simulink model "ControlloRobusto"  (R2021a)
settings: Solver=VariableStepAuto  StartTime=0.0  StopTime=50  RelTol=1e-3
values from neighbouring files (symbols this model uses):
  KD = kdi*eye(4)    [traiettoria.m]
  Kd = 200*diag([1 1 1 1])    [traiettoria.m]
  KP = kpi*eye(4)    [traiettoria.m]
  q0 = scara.ikine(T0, 'mask', [1 1 1 1 0 0])    [pseudo_traiettoria.m]    (also in traiettoria.m)
  Tc = 0.001    [pseudo_traiettoria.m]    (also in traiettoria.m)
undefined symbols (not defined in the file or in its folder): D, DiscIntNeverNeededParam, Kp, Q
settings Model: Creator=Ciro  LastModifiedBy=Ciro

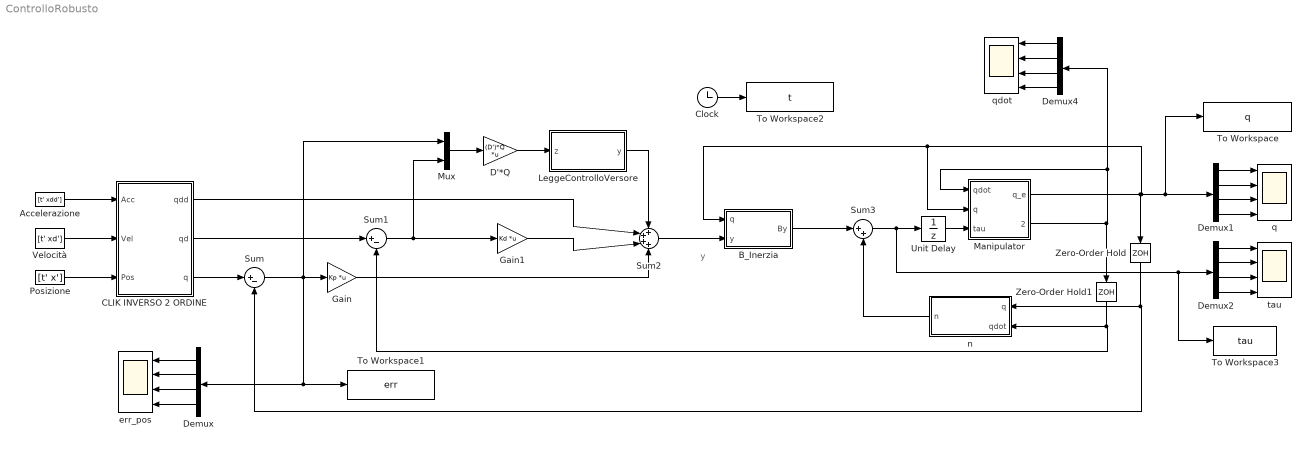
== system ControlloRobusto ==
  note: y
  Accelerazione : FromWorkspace  VariableName=[t' xdd']  SampleTime=Tc  OutputAfterFinalValue=Holding final value
  B_Inerzia : MATLAB Function  TreatAsAtomicUnit=on
  CLIK INVERSO 2 ORDINE : Subsystem
  Clock : Clock
  D'*Q : Gain  Gain=(D')*Q  Multiplication=Matrix(K*u)
  Demux{,1..2,4} (4 alike) : Demux
  Gain : Gain  Gain=Kp  Multiplication=Matrix(K*u)
  Gain1 : Gain  Gain=Kd  Multiplication=Matrix(K*u)
  LeggeControlloVersore : MATLAB Function  TreatAsAtomicUnit=on
  Manipulator : Subsystem
  Mux : Mux  Inputs=2
  Posizione : FromWorkspace  VariableName=[t' x']  SampleTime=Tc  OutputAfterFinalValue=Holding final value
  Sum : Sum  Inputs=|+-
  Sum1 : Sum  Inputs=|+-
  Sum2 : Sum  Inputs=++++
  Sum3 : Sum  Inputs=|++
  To Workspace : ToWorkspace  VariableName=q  SampleTime=-1
      settings: Save2DSignal=2-D array (concatenate along first dimension)
  To Workspace1 : ToWorkspace  VariableName=err  SampleTime=-1
      settings: Save2DSignal=2-D array (concatenate along first dimension)
  To Workspace2 : ToWorkspace  VariableName=t  SampleTime=-1
      settings: Save2DSignal=2-D array (concatenate along first dimension)
  To Workspace3 : ToWorkspace  VariableName=tau  SampleTime=-1
      settings: Save2DSignal=2-D array (concatenate along first dimension)
  Unit Delay : UnitDelay  SampleTime=Tc  HasFrameUpgradeWarning=on
  Velocità : FromWorkspace  VariableName=[t' xd']  SampleTime=Tc  OutputAfterFinalValue=Holding final value
  Zero-Order Hold : ZeroOrderHold  SampleTime=Tc
  Zero-Order Hold1 : ZeroOrderHold  SampleTime=Tc
  err_pos : Scope  NumInputPorts=4
  n : MATLAB Function  TreatAsAtomicUnit=on
  q : Scope  NumInputPorts=4
  qdot : Scope  NumInputPorts=4
  tau : Scope  NumInputPorts=4
  wires:
  Accelerazione/1 -> CLIK INVERSO 2 ORDINE/1(Acc)
  Velocità/1 -> CLIK INVERSO 2 ORDINE/2(Vel)
  Posizione/1 -> CLIK INVERSO 2 ORDINE/3(Pos)
  Sum/1 -> Mux/1, Gain/1, To Workspace1/1, Demux/1
  Sum1/1 -> Mux/2, Gain1/1
  B_Inerzia/1(By) -> Sum3/1
  CLIK INVERSO 2 ORDINE/3(q) -> Sum/1
  CLIK INVERSO 2 ORDINE/2(qd) -> Sum1/1
  n/1(n) -> Sum3/2
  Sum3/1 -> Unit Delay/1, To Workspace3/1, Demux2/1
  Gain1/1 -> Sum2/3
  CLIK INVERSO 2 ORDINE/1(qdd) -> Sum2/2
  Demux/1 -> err_pos/1
  Demux/2 -> err_pos/2
  Demux/3 -> err_pos/3
  Demux/4 -> err_pos/4
  Demux1/1 -> q/1
  Demux1/2 -> q/2
  Demux1/3 -> q/3
  Demux1/4 -> q/4
  Demux2/4 -> tau/4
  Demux2/3 -> tau/3
  Demux2/2 -> tau/2
  Demux2/1 -> tau/1
  LeggeControlloVersore/1(y) -> Sum2/1
  Mux/1 -> D'*Q/1
  D'*Q/1 -> LeggeControlloVersore/1(z)
  Demux4/4 -> qdot/4
  Demux4/3 -> qdot/3
  Demux4/2 -> qdot/2
  Demux4/1 -> qdot/1
  Gain/1 -> Sum2/4
  Manipulator/1(q_e) -> Demux1/1, To Workspace/1, B_Inerzia/1(q), Manipulator/2(q), Zero-Order Hold/1
  Manipulator/2(qdot_e) -> Demux4/1, Manipulator/1(qdot), Zero-Order Hold1/1
  Zero-Order Hold/1 -> Sum/2, n/1(q)
  Zero-Order Hold1/1 -> Sum1/2, n/2(qdot)
  Sum2/1 -> B_Inerzia/2(y)
  Unit Delay/1 -> Manipulator/3(tau)
  Clock/1 -> To Workspace2/1

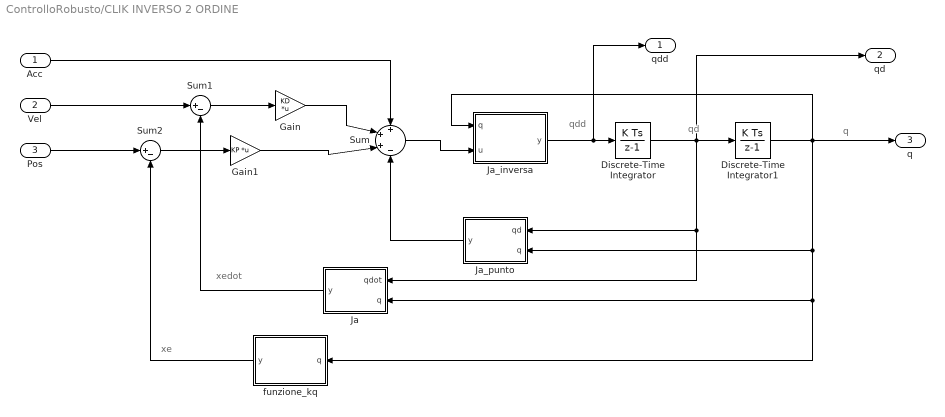
== system ControlloRobusto/CLIK INVERSO 2 ORDINE ==
  note: qdd
  note: xedot
  note: xe
  note: qd
  note: q
  Acc : Inport
  Vel : Inport  Port=2
  Pos : Inport  Port=3
  Discrete-Time Integrator : DiscreteIntegrator  InitialCondition=[0; 0; 0; 0]  SampleTime=Tc  ICPrevOutput=DiscIntNeverNeededParam  ICPrevScaledInput=DiscIntNeverNeededParam
  Discrete-Time Integrator1 : DiscreteIntegrator  InitialCondition=q0  SampleTime=Tc  ICPrevOutput=DiscIntNeverNeededParam  ICPrevScaledInput=DiscIntNeverNeededParam
  Gain : Gain  Gain=KD  Multiplication=Matrix(K*u)
  Gain1 : Gain  Gain=KP  Multiplication=Matrix(K*u)
  Ja : MATLAB Function  TreatAsAtomicUnit=on
  Ja_inversa : MATLAB Function  TreatAsAtomicUnit=on
  Ja_punto : MATLAB Function  TreatAsAtomicUnit=on
  Sum : Sum  Inputs=+++-
  Sum1 : Sum  Inputs=|+-
  Sum2 : Sum  Inputs=|+-
  funzione_kq : MATLAB Function  TreatAsAtomicUnit=on
  qdd : Outport
  qd : Outport  Port=2
  q : Outport  Port=3
  wires:
  Gain1/1 -> Sum/3
  Discrete-Time Integrator1/1 -> q/1, Ja_punto/2(q), Ja/2(q), funzione_kq/1(q), Ja_inversa/1(q)
  Ja_punto/1(y) -> Sum/4
  Pos/1 -> Sum2/1
  Sum/1 -> Ja_inversa/2(u)
  Gain/1 -> Sum/2
  Sum2/1 -> Gain1/1
  funzione_kq/1(y) -> Sum2/2
  Ja/1(y) -> Sum1/2
  Sum1/1 -> Gain/1
  Vel/1 -> Sum1/1
  Acc/1 -> Sum/1
  Discrete-Time Integrator/1 -> qd/1, Ja_punto/1(qd), Ja/1(qdot), Discrete-Time Integrator1/1
  Ja_inversa/1(y) -> qdd/1, Discrete-Time Integrator/1

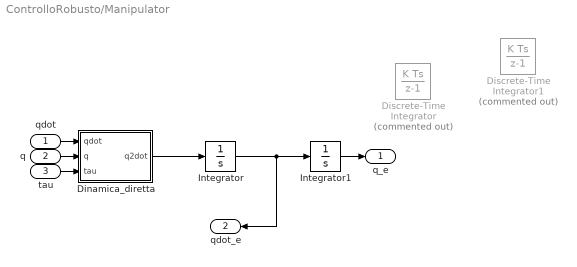
== system ControlloRobusto/Manipulator ==
  qdot : Inport
  q : Inport  Port=2
  tau : Inport  Port=3
  Dinamica_diretta : MATLAB Function  TreatAsAtomicUnit=on
  Discrete-Time Integrator : DiscreteIntegrator  Commented=on  InitialCondition=[0; 0; 0; 0]  SampleTime=Tc  ICPrevOutput=DiscIntNeverNeededParam  ICPrevScaledInput=DiscIntNeverNeededParam
  Discrete-Time Integrator1 : DiscreteIntegrator  Commented=on  InitialCondition=q0  SampleTime=Tc  ICPrevOutput=DiscIntNeverNeededParam  ICPrevScaledInput=DiscIntNeverNeededParam
  Integrator : Integrator  InitialCondition=[0; 0; 0; 0]
  Integrator1 : Integrator  InitialCondition=q0
  q_e : Outport
  qdot_e : Outport  Port=2
  wires:
  tau/1 -> Dinamica_diretta/3(tau)
  qdot/1 -> Dinamica_diretta/1(qdot)
  q/1 -> Dinamica_diretta/2(q)
  Integrator1/1 -> q_e/1
  Integrator/1 -> Integrator1/1, qdot_e/1
  Dinamica_diretta/1(q2dot) -> Integrator/1

== matlab function ControlloRobusto/CLIK INVERSO 2 ORDINE/Ja_inversa ==
  data: q input; u input; y output
function y = fcn(q, u)
J = [ -0.5*(sin(q(1))+sin(q(1)+q(2))) -0.5*sin(q(1)+q(2))  0  0;
       0.5*(cos(q(1))+cos(q(1)+q(2)))  0.5*cos(q(1)+q(2))  0  0;
       0                               0                  -1  0;
       1                               1                   0 -1];
y = inv(J)*u;

== matlab function ControlloRobusto/CLIK INVERSO 2 ORDINE/Ja ==
  data: qdot input; q input; y output
function y = fcn(qdot,q)
J = [ -0.5*(sin(q(1))+sin(q(1)+q(2))) -0.5*sin(q(1)+q(2))  0  0;
       0.5*(cos(q(1))+cos(q(1)+q(2)))  0.5*cos(q(1)+q(2))  0  0;
       0                               0                  -1  0;
       1                               1                   0 -1];
y = J*qdot;

== matlab function ControlloRobusto/CLIK INVERSO 2 ORDINE/Ja_punto ==
  data: qd input; q input; y output
function y = fcn(qd,q)
Jpunto = [ -0.5*(cos(q(1))*qd(1) + cos(q(1)+q(2))*(qd(1)+qd(2)))    -0.5*cos(q(1)+q(2))*(qd(1)+qd(2))  0  0;
           -0.5*(sin(q(1))*qd(1) + sin(q(1)+q(2))*(qd(1)+qd(2)))    -0.5*sin(q(1)+q(2))*(qd(1)+qd(2))  0  0;
           0                                                        0                                  0  0;
           0                                                        0                                  0  0];
y = Jpunto*qd;

== matlab function ControlloRobusto/Manipulator/Dinamica_diretta ==
  data: qdot input; q input; tau input; q2dot output
function q2dot = fcn(qdot,q,tau)

a1 = 0.5;
a2 = 0.5;

%% Dinamica

%masse
ml1 = 25;
ml2 = 25;
ml3 = 10;

%posizioni baricentro
L1 = 0.25;
L2 = 0.25;

%inerzie di massa bracci
Il1 = 5;
Il2 = 5;
Il4 = 1;

%rapporti di trasmissione;
Kr1 = 1;
Kr2 = 1;
Kr3 = 50;
Kr4 = 20;

%inerzie motori
Im1 = 0.02;
Im2 = 0.02;
Im3 = 0.005;
Im4 = 0.001;

%attriti dei motori
Fm1 = 0.0001;
Fm2 = 0.0001;
Fm3 = 0.01;
Fm4 = 0.005;

load = 5;

q2 = q(2);
q1d = qdot(1);
q2d = qdot(2);
q3d = qdot(3);
q4d = qdot(4);

B=[Il1 + Il2 + Il4 + Im2 + Im3 + Im4 + Im1*Kr1^2 + L1^2*ml1 + L2^2*ml2 + a1^2*load + a2^2*load + a1^2*ml2 + a1^2*ml3 + a2^2*ml3 + 2*L2*a1*ml2*cos(q2) + 2*a1*a2*load*cos(q2) + 2*a1*a2*ml3*cos(q2), Il2 + Il4 + Im3 + Im4 + L2^2*ml2 + a2^2*load + a2^2*ml3 + L2*a1*ml2*cos(q2) + a1*a2*load*cos(q2) + a1*a2*ml3*cos(q2),                      0,        - Il4 - Im4;
                                                                           Il2 + Il4 + Im3 + Im4 + L2^2*ml2 + a2^2*load + a2^2*ml3 + L2*a1*ml2*cos(q2) + a1*a2*load*cos(q2) + a1*a2*ml3*cos(q2),                                                  Il2 + Il4 + Im3 + Im4 + Im2*Kr2^2 + L2^2*ml2 + a2^2*load + a2^2*ml3,                      0,           - Il4 - Im4;
                                                                                                                                                                                              0,                                                                                                                    0, Im3*Kr3^2 + load + ml3,                     0;
                                                                                                                                                                                    - Il4 - Im4,                                                                                                          - Il4 - Im4,                      0, Im4*Kr4^2 + Il4 + Im4];
C = [-a1*q2d*sin(q2)*(L2*ml2 + a2*load + a2*ml3), -a1*sin(q2)*(q1d + q2d)*(L2*ml2 + a2*load + a2*ml3), 0, 0;
 a1*q1d*sin(q2)*(L2*ml2 + a2*load + a2*ml3),                                                   0, 0, 0;
                                          0,                                                   0, 0, 0;
                                          0,                                                   0, 0, 0];


Fv = [-Fm1*q1d*abs(Kr1)^2; -Fm2*q2d*abs(Kr2)^2; -Fm3*q3d*abs(Kr3)^2; -Fm4*q4d*abs(Kr4)^2];
g = [0, 0, - 9.81*load - 9.81*ml3, 0]';
tau_primo = C*qdot+Fv+g;

q2dot = inv(B)*(tau-tau_primo);

== matlab function ControlloRobusto/B_Inerzia ==
  data: q input; By output; y input
function By = B_hat(q,y)

a1 = 0.5;
a2 = 0.5;

%masse
ml1 = 25;
ml2 = 25;
ml3 = 10;

%posizioni baricentro
L1 = 0.25;
L2 = 0.25;

%inerzie di massa bracci
Il1 = 5;
Il2 = 5;
Il4 = 1;

%rapporti di trasmissione;
Kr1 = 1;
Kr2 = 1;
Kr3 = 50;
Kr4 = 20;

%inerzie motori
Im1 = 0.02;
Im2 = 0.02;
Im3 = 0.005;
Im4 = 0.001;

load = 5;

q2 = q(2);

% Bi=[Il1 + Il2 + Il4 + Im2 + Im3 + Im4 + Im1*Kr1^2 + L1^2*ml1 + L2^2*ml2 + a1^2*load + a2^2*load + a1^2*ml2 + a1^2*ml3 + a2^2*ml3 + 2*L2*a1*ml2*cos(q2) + 2*a1*a2*load*cos(q2) + 2*a1*a2*ml3*cos(q2), Il2 + Il4 + Im3 + Im4 + L2^2*ml2 + a2^2*load + a2^2*ml3 + L2*a1*ml2*cos(q2) + a1*a2*load*cos(q2) + a1*a2*ml3*cos(q2),                      0,        - Il4 - Im4;
%                                                                            Il2 + Il4 + Im3 + Im4 + L2^2*ml2 + a2^2*load + a2^2*ml3 + L2*a1*ml2*cos(q2) + a1*a2*load*cos(q2) + a1*a2*ml3*cos(q2),                                                  Il2 + Il4 + Im3 + Im4 + Im2*Kr2^2 + L2^2*ml2 + a2^2*load + a2^2*ml3,                      0,           - Il4 - Im4;
%                                                                                                                                                                                               0,                                                                                                                    0, Im3*Kr3^2 + load + ml3,                     0;
%                                                                                                                                                                                     - Il4 - Im4,                                                                                                          - Il4 - Im4,                      0, Im4*Kr4^2 + Il4 + Im4];

B=[Il1 + Il2 + Il4 + Im2 + Im3 + Im4 + Im1*Kr1^2 + L1^2*ml1 + L2^2*ml2 + a1^2*load + a2^2*load + a1^2*ml2 + a1^2*ml3 + a2^2*ml3 + 2*L2*a1*ml2*cos(q2) + 2*a1*a2*load*cos(q2) + 2*a1*a2*ml3*cos(q2),                                                                           0,                      0,                     0;
                                                                                                                                                                                                 0,         Il2 + Il4 + Im3 + Im4 + Im2*Kr2^2 + L2^2*ml2 + a2^2*load + a2^2*ml3,                      0,                     0;
                                                                                                                                                                                                 0,                                                                           0, Im3*Kr3^2 + load + ml3,                     0;
                                                                                                                                                                                                 0,                                                                           0,                      0, Im4*Kr4^2 + Il4 + Im4];

By = B*y;

== matlab function ControlloRobusto/n ==
  data: q input; n output; qdot input
function n = n_hat(q,qdot)
a1 = 0.5;
a2 = 0.5;

%% Dinamica

%masse
ml2 = 25;
ml3 = 10;

%posizioni baricentro
L2 = 0.25;

%rapporti di trasmissione;
Kr1 = 1;
Kr2 = 1;
Kr3 = 50;
Kr4 = 20;

%attriti dei motori
Fm1 = 0.0001;
Fm2 = 0.0001;
Fm3 = 0.01;
Fm4 = 0.005;

load = 5;

q2 = q(2);
q1d = qdot(1);
q2d = qdot(2);
q3d = qdot(3);
q4d = qdot(4);

% C = [-a1*q2d*sin(q2)*(L2*ml2 + a2*load + a2*ml3), -a1*sin(q2)*(q1d + q2d)*(L2*ml2 + a2*load + a2*ml3), 0, 0;
%       a1*q1d*sin(q2)*(L2*ml2 + a2*load + a2*ml3),                                                   0, 0, 0;
%                                                0,                                                   0, 0, 0;
%                                                0,                                                   0, 0, 0];


%Fv = [-Fm1*q1d*abs(Kr1)^2; -Fm2*q2d*abs(Kr2)^2; -Fm3*q3d*abs(Kr3)^2; -Fm4*q4d*abs(Kr4)^2];
g = [0, 0, - 9.81*load - 9.81*ml3, 0]';
n = g;

== matlab function ControlloRobusto/LeggeControlloVersore ==
  data: z input; y output
function y = rhoVersore(z)
versore = z/norm(z);
rho = 4;
epsilon = 0.14;
if norm(z)>=epsilon
   rovers = rho*versore;
    
else
    rovers = rho*z/epsilon;
end
    
y = rovers;

== matlab function ControlloRobusto/CLIK INVERSO 2 ORDINE/funzione_kq ==
  data: q input; y output
function y = fcn(q)

xe = [0.5*(cos(q(1))+cos(q(1)+q(2)));
      0.5*(sin(q(1))+sin(q(1)+q(2)));
      0.8-q(3);
      q(1)+q(2)-q(4)];

y = xe;
